simulink model "tvc_PID_workingmodel"  (R2024a)
settings: Solver=VariableStepAuto  StartTime=0.0  StopTime=10
undefined symbols (not defined in the file): X, Y, Z
libraries: sm_lib x45, nesl_utility x26, slpidlib x6, simulink_extras x3
(part 1 of 3)
settings Model: Creator=MichaelGerits  LastModifiedBy=MichaelGerits
settings ExplorerConfigSet: InternalSimMechanicsExplorerSettings="<ExplorerConfiguration><canonicalview>default</canonicalview><AnimationSetting><BasePlaybackSpeed>1.0</BasePlaybackSpeed><PlaybackSpeedFactor>1.0</PlaybackSpeedFactor></AnimationSetting><TilePanel><TileInfo><Tiles Columns=\"1\" Count=\"1\" Rows=\"1\"><Column Weight=\"1\"/><Row Weight=\"1\"/><Tile Height=\"1\" Width=\"1\" X=\"0\" Y=\"0\"/></Tiles></TileInfo><SceneInfo><SceneViewer><BGColor><R>0.800000011920928955</R><G>0.800000011920928955</G><B>0.800000011920928955</B></BGColor><Camera><DoPerspective>on</DoPerspective><Position><X>12.244083106589569</X><Y>-12.2640491877965125</Y><Z>14.9754935505138143</Z></Position><Center><X>-0.355803163378928033</X><Y>0.335837082171984491</Y><Z>2.37560728054531722</Z></Center><Up><X>-0.408248290463863073</X><Y>0.408248290463863073</Y><Z>0.816496580927726145</Z></Up><ViewLimDist>1</ViewLimDist><YLim>0.466307658154998583</YLim><XLim>0.334171826028237029</XLim></Camera></SceneViewer></SceneInfo></TilePanel><MechEditorPanel><Cameras><Camera><Id>Camera1</Id><Value><Name>follow pendulum</Name><NativeCamera><PositionTrackingFeature>single_axis_inverted_pendulum.pendulum.Frame1</PositionTrackingFeature><CenterTrackingFeature/><UpVectorTrackingFeature/><CenterTrackingOrigin>off</CenterTrackingOrigin><CenterTrackingDirection>+Y</CenterTrackingDirection><UpVectorTrackingDirection>+X</UpVectorTrackingDirection></NativeCamera></Value></Camera></Cameras><GfxPanelCameraMap><MapElement CameraMLId=\"Camera1\" GfxPanelIndex=\"0\"/></GfxPanelCameraMap><VideoCreator><PlaybackSpeedRatio>1.0</PlaybackSpeedRatio><FrameRate>30</FrameRate><VideoFormat>Motion JPEG AVI</VideoFormat><FrameSize>auto</FrameSize></VideoCreator></MechEditorPanel></ExplorerConfiguration>"

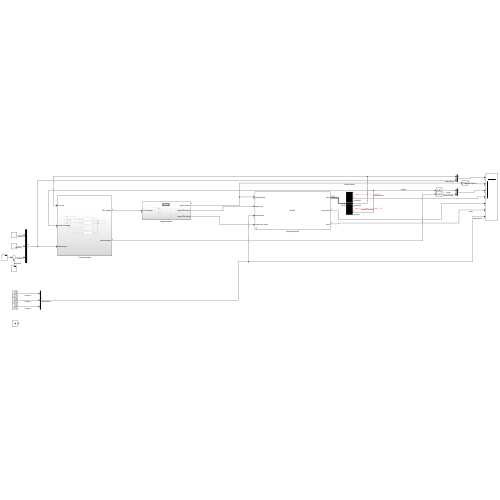
[thumbnail: Simulink's stored preview of the top-level diagram]
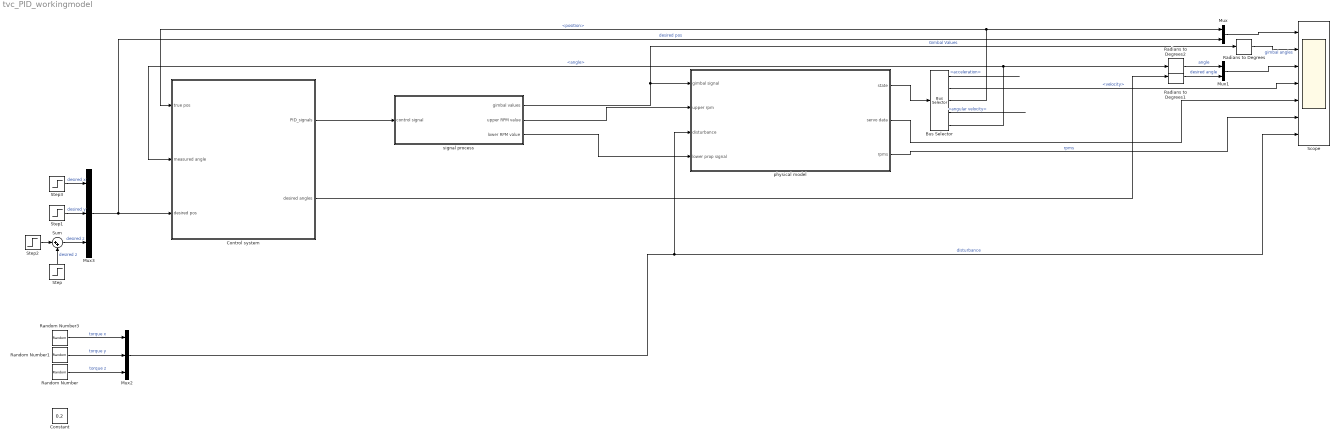
== system tvc_PID_workingmodel ==
  Bus Selector : BusSelector  OutputSignals=acceleration,velocity,position,angular velocity,angle
  Constant : Constant  Value=0.2
  Control system : Subsystem
  Mux : Mux  Inputs=2
  Mux1 : Mux  Inputs=2
  Mux2 : Mux  Inputs=3
  Mux3 : Mux  Inputs=3
  Radians to Degrees : simulink_extras/Transformations/Radians to Degrees
  Radians to Degrees1 : simulink_extras/Transformations/Radians to Degrees
  Radians to Degrees2 : simulink_extras/Transformations/Radians to Degrees
  Random Number : RandomNumber  Variance=0  SampleTime=2
  Random Number1 : RandomNumber  Variance=0  SampleTime=0.5
  Random Number3 : RandomNumber  Variance=0  Seed=0.25  SampleTime=2
  Scope : Scope  NumInputPorts=7
  Step : Step  Time=25  After=0  SampleTime=0
  Step1 : Step  Time=0.5  After=0  SampleTime=0
  Step2 : Step  After=0  SampleTime=0
  Step3 : Step  Time=0.5  After=0  SampleTime=0
  Sum : Sum  Inputs=|++
  physical model : Subsystem  mask{D=0.2286, m=0.01, Kt=4.65e-5, Kq=0.000614, RPM_rate=6000, RPM_lim=9000, Servo_acc=1*10e3, Servo_rate=250, Servo_lim=20}
      mask prompts: D "Prop Diameter:"; m "Prop Mass"; Kt "thrust coefficient:"; Kq "Torque Coefficient"; RPM_rate "RPM rate:"; RPM_lim "RPM limit:"; Servo_acc "Servo acceleration:"; Servo_rate "Gimbal rate:"; Servo_lim "Gimbal Limit:"
      mask Display: disp('Model');
  signal process : Subsystem
  wires:
  physical model/1(state) -> Bus Selector/1
  Random Number3/1 -> Mux2/1  "torque x"
  Random Number1/1 -> Mux2/2  "torque y"
  Control system/1(PID_signals) -> signal process/1(control signal)
  Step3/1 -> Mux3/1  "desired x"
  Step1/1 -> Mux3/2  "desired y"
  Sum/1 -> Mux3/3  "desired z"
  Mux3/1 -> Mux/2, Control system/3(desired pos)  "desired pos"
  Mux2/1 -> Scope/7, physical model/3(disturbance)  "disturbance"
  Bus Selector/5 -> Control system/2(measured angle), Radians to Degrees2/1  "<angle>"
  Bus Selector/4 -> ?  "<angular velocity>"
  Bus Selector/3 -> Mux/1, Control system/1(true pos)  "<position>"
  Bus Selector/2 -> Scope/4  "<velocity>"
  Bus Selector/1 -> ?  "<acceleration>"
  signal process/1(gimbal values) -> Radians to Degrees/1, physical model/1(gimbal signal)  "Gimbal Values"
  Control system/2(desired angles) -> Radians to Degrees1/1
  Mux/1 -> Scope/1
  Random Number/1 -> Mux2/3  "torque z"
  Step/1 -> Sum/2  "desired z"
  Step2/1 -> Sum/1
  physical model/2(servo data) -> Scope/5
  signal process/2(upper RPM value) -> physical model/2(upper rpm)
  Radians to Degrees/1 -> Scope/2  "gimbal angles"
  Mux1/1 -> Scope/3
  Radians to Degrees2/1 -> Mux1/1  "angle"
  Radians to Degrees1/1 -> Mux1/2  "desired angle"
  physical model/3(rpms) -> Scope/6  "rpms"
  signal process/3(lower RPM value) -> physical model/4(lower prop signal)

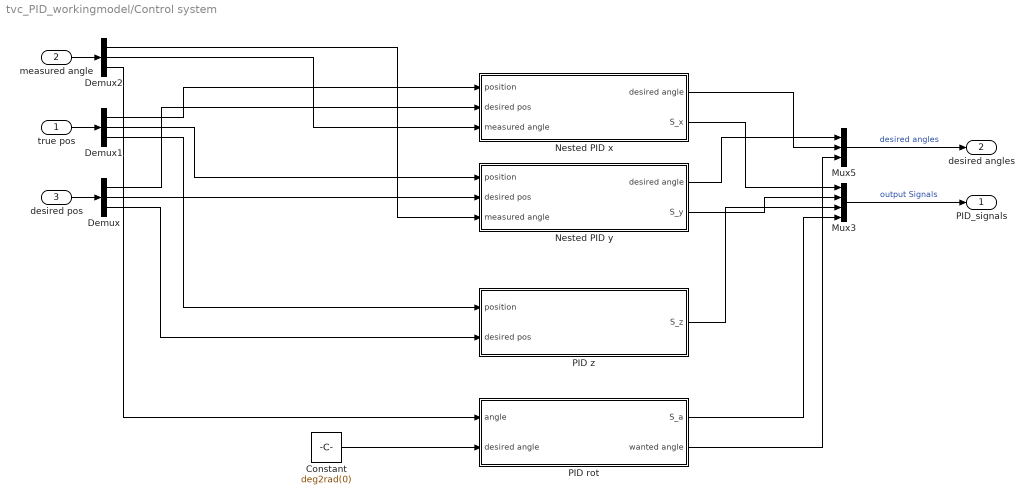
== system tvc_PID_workingmodel/Control system ==
  true pos : Inport
  measured angle : Inport  Port=2
  desired pos : Inport  Port=3
  " PID rot" : Subsystem
  " PID z" : Subsystem
  Constant : Constant  Value=deg2rad(0)
  Demux : Demux  Outputs=3
  Demux1 : Demux  Outputs=3
  Demux2 : Demux  Outputs=3
  Mux3 : Mux
  Mux5 : Mux  Inputs=3
  Nested PID x : Subsystem
  Nested PID y : Subsystem
  PID_signals : Outport
  desired angles : Outport  Port=2
  wires:
  Mux5/1 -> desired angles/1  "desired angles"
  " PID z"/1(S_z) -> Mux3/3
  Nested PID x/1(desired angle) -> Mux5/2
  Nested PID y/1(desired angle) -> Mux5/1
  Nested PID y/2(S_y) -> Mux3/2
  Mux3/1 -> PID_signals/1  "output Signals"
  Nested PID x/2(S_x) -> Mux3/1
  Demux2/1 -> Nested PID y/3(measured angle)
  Demux2/2 -> Nested PID x/3(measured angle)
  Demux/2 -> Nested PID y/2(desired pos)
  Demux/3 -> " PID z"/2(desired pos)
  desired pos/1 -> Demux/1
  Demux/1 -> Nested PID x/2(desired pos)
  true pos/1 -> Demux1/1
  Demux1/1 -> Nested PID x/1(position)
  Demux1/2 -> Nested PID y/1(position)
  Demux1/3 -> " PID z"/1(position)
  measured angle/1 -> Demux2/1
  " PID rot"/1(S_a) -> Mux3/4
  Demux2/3 -> " PID rot"/1(angle)
  Constant/1 -> " PID rot"/2(desired angle)
  " PID rot"/2(wanted angle) -> Mux5/3
